simulink model "uavPackageDelivery_3UAV_photo3D_test"  (R2026a)
settings: Solver=VariableStepAuto  StopTime=20  FixedStep=.005  EnableMultiTasking=on
undefined symbols (not defined in the file or in its folder): baseMission, Newton, oaMission, Raphson, uavIC_latLon, UAVSampleTime
libraries: robotcorelib x3, uavalgslib x3, robotalgslib x3, simulink x2
(part 1 of 2)
settings Model: DataDictionary=uavPackageDeliveryDataDict.sldd  ModifiedByFormat=The MathWorks, Inc.  PauseTimes=77  Creator=The MathWorks, Inc.  LastModifiedBy=The MathWorks, Inc.
settings OptimizationCC: DefaultUnderspecifiedDataType=single  PassReuseOutputArgsThreshold=0.0
settings DebuggingCC: ParameterPrecisionLossMsg=none
settings HardwareCC: ProdHWDeviceType=Generic->Unspecified (assume 32-bit Generic)
settings RTWCC: GenerateReport=on  LaunchReport=on

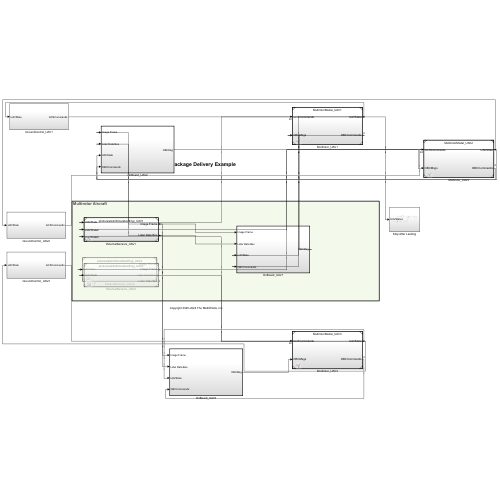
[thumbnail: Simulink's stored preview of the top-level diagram]
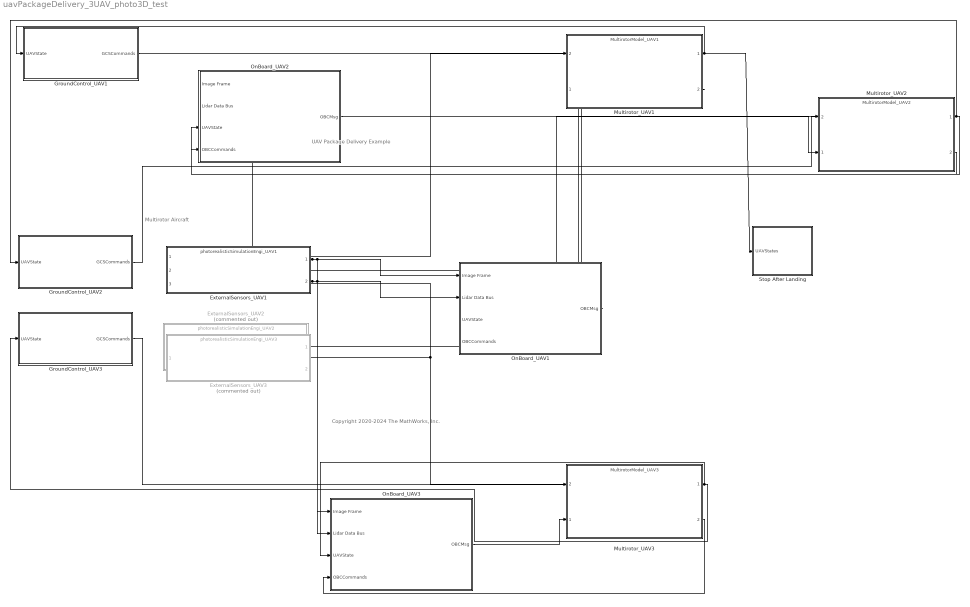
== system uavPackageDelivery_3UAV_photo3D_test ==
  note: Multirotor Aircraft
  note: UAV Package Delivery Example
  note: Copyright 2020-2024 The MathWorks, Inc.
  ExternalSensors_UAV1 : ModelReference  ModelNameDialog=photorealisticSimulationEngi_UAV1  SimulationMode=Normal  ModelReferenceVersion=12.27
  ExternalSensors_UAV2 : ModelReference  Commented=on  ModelNameDialog=photorealisticSimulationEngi_UAV2  SimulationMode=Normal  ModelReferenceVersion=12.1
  ExternalSensors_UAV3 : ModelReference  Commented=on  ModelNameDialog=photorealisticSimulationEngi_UAV3  SimulationMode=Normal  ModelReferenceVersion=12.1
  GroundControl_UAV1 : Subsystem
  GroundControl_UAV2 : Subsystem
  GroundControl_UAV3 : Subsystem
  Multirotor_UAV1 : ModelReference  ModelNameDialog=MultirotorModel_UAV1  SimulationMode=Normal  ModelReferenceVersion=13.15
      settings: PortSchema="{\"entries\":[{\"content\":{\"sides\":[{\"content\":{\"connectorIds\":[\"In2\",\"In1\"]},\"type\":\"ConnectorPlacement.EquallySpacedRectSide\",\"uuid\":\"abf53b88-b4c0-4cc3-bb4c-819ba68ade90\"},{\"content\":{\"connectorIds\":[\"Out1\",\"Out2\"],\"side\":\"RIGHT\"},\"type\":\"ConnectorPlacement.EquallySpacedRectSide\",\"uuid\":\"f1944fd3-3680-4558-bd6a-ffb0187ae725\"},{\"content\":{\"connectorIds\":[],\"side\":\"TOP\"},\"type\":\"ConnectorPlacement.EquallySpacedRectSide\",\"uuid\":\"7f686bac-a1b4-4e90-bc1f-e4dd6e8ae5c6\"}]},\"type\":\"ConnectorPlacement.EquallySpacedConnector\",\"uuid\":\"3f45c06a-90ee-44cf-add7-da13163a6845\"}],\"packageUris\":[\"http://schema.mathworks.com/mf0/Connector/19700101\"],\"version\":\"1.0\"}"
  Multirotor_UAV2 : ModelReference  ModelNameDialog=MultirotorModel_UAV2  SimulationMode=Normal  ModelReferenceVersion=13.16
      settings: PortSchema="{\"entries\":[{\"content\":{\"sides\":[{\"content\":{\"connectorIds\":[\"In2\",\"In1\"]},\"type\":\"ConnectorPlacement.EquallySpacedRectSide\",\"uuid\":\"abf53b88-b4c0-4cc3-bb4c-819ba68ade90\"},{\"content\":{\"connectorIds\":[\"Out1\",\"Out2\"],\"side\":\"RIGHT\"},\"type\":\"ConnectorPlacement.EquallySpacedRectSide\",\"uuid\":\"f1944fd3-3680-4558-bd6a-ffb0187ae725\"},{\"content\":{\"connectorIds\":[],\"side\":\"TOP\"},\"type\":\"ConnectorPlacement.EquallySpacedRectSide\",\"uuid\":\"7f686bac-a1b4-4e90-bc1f-e4dd6e8ae5c6\"}]},\"type\":\"ConnectorPlacement.EquallySpacedConnector\",\"uuid\":\"3f45c06a-90ee-44cf-add7-da13163a6845\"}],\"packageUris\":[\"http://schema.mathworks.com/mf0/Connector/19700101\"],\"version\":\"1.0\"}"
  Multirotor_UAV3 : ModelReference  ModelNameDialog=MultirotorModel_UAV3  SimulationMode=Normal  ModelReferenceVersion=13.16
      settings: PortSchema="{\"entries\":[{\"content\":{\"sides\":[{\"content\":{\"connectorIds\":[\"In2\",\"In1\"]},\"type\":\"ConnectorPlacement.EquallySpacedRectSide\",\"uuid\":\"abf53b88-b4c0-4cc3-bb4c-819ba68ade90\"},{\"content\":{\"connectorIds\":[\"Out1\",\"Out2\"],\"side\":\"RIGHT\"},\"type\":\"ConnectorPlacement.EquallySpacedRectSide\",\"uuid\":\"f1944fd3-3680-4558-bd6a-ffb0187ae725\"},{\"content\":{\"connectorIds\":[],\"side\":\"TOP\"},\"type\":\"ConnectorPlacement.EquallySpacedRectSide\",\"uuid\":\"7f686bac-a1b4-4e90-bc1f-e4dd6e8ae5c6\"}]},\"type\":\"ConnectorPlacement.EquallySpacedConnector\",\"uuid\":\"3f45c06a-90ee-44cf-add7-da13163a6845\"}],\"packageUris\":[\"http://schema.mathworks.com/mf0/Connector/19700101\"],\"version\":\"1.0\"}"
  OnBoard_UAV1 : Subsystem  TreatAsAtomicUnit=on
  OnBoard_UAV2 : Subsystem  TreatAsAtomicUnit=on
  OnBoard_UAV3 : Subsystem  TreatAsAtomicUnit=on
  Stop After Landing : Subsystem
  wires:
  GroundControl_UAV1/1(GCSCommands) -> Multirotor_UAV1/2
  Multirotor_UAV1/1 -> OnBoard_UAV1/3(UAVState), ExternalSensors_UAV1/1, GroundControl_UAV1/1(UAVState), Stop After Landing/1(UAVStates)
  Multirotor_UAV1/2 -> OnBoard_UAV1/4(OBCCommands)
  OnBoard_UAV1/1(OBCMsg) -> Multirotor_UAV1/1
  GroundControl_UAV2/1(GCSCommands) -> Multirotor_UAV2/2
  Multirotor_UAV2/1 -> ExternalSensors_UAV2/1, ExternalSensors_UAV1/2, GroundControl_UAV2/1(UAVState), OnBoard_UAV2/3(UAVState)
  Multirotor_UAV2/2 -> OnBoard_UAV2/4(OBCCommands)
  OnBoard_UAV2/1(OBCMsg) -> Multirotor_UAV2/1
  GroundControl_UAV3/1(GCSCommands) -> Multirotor_UAV3/2
  Multirotor_UAV3/1 -> ExternalSensors_UAV3/1, ExternalSensors_UAV1/3, GroundControl_UAV3/1(UAVState), OnBoard_UAV3/3(UAVState)
  Multirotor_UAV3/2 -> OnBoard_UAV3/4(OBCCommands)
  OnBoard_UAV3/1(OBCMsg) -> Multirotor_UAV3/1
  ExternalSensors_UAV1/1 -> OnBoard_UAV1/1(Image Frame), OnBoard_UAV3/1(Image Frame), OnBoard_UAV2/1(Image Frame)
  ExternalSensors_UAV1/2 -> OnBoard_UAV1/2("Lidar Data Bus "), OnBoard_UAV3/2("Lidar Data Bus "), OnBoard_UAV2/2("Lidar Data Bus ")

== system uavPackageDelivery_3UAV_photo3D_test/GroundControl_UAV1 ==
  UAVState : Inport  OutDataTypeStr=Bus: uavStateBus
  Get Flight Mission : Subsystem  Variant=on
  Rate Transition : RateTransition  OutPortSampleTime=UAVSampleTime*4
  GCSCommands : Outport
  wires:
  UAVState/1 -> Rate Transition/1
  Get Flight Mission/1("Mission ") -> GCSCommands/1
  Rate Transition/1 -> Get Flight Mission/1(UAVState)

== system uavPackageDelivery_3UAV_photo3D_test/GroundControl_UAV2 ==
  UAVState : Inport  OutDataTypeStr=Bus: uavStateBus
  Get Flight Mission : Subsystem  Variant=on
  Rate Transition : RateTransition  OutPortSampleTime=UAVSampleTime*4
  GCSCommands : Outport
  wires:
  UAVState/1 -> Rate Transition/1
  Get Flight Mission/1("Mission ") -> GCSCommands/1
  Rate Transition/1 -> Get Flight Mission/1(UAVState)

== system uavPackageDelivery_3UAV_photo3D_test/GroundControl_UAV3 ==
  UAVState : Inport  OutDataTypeStr=Bus: uavStateBus
  Get Flight Mission : Subsystem  Variant=on
  Rate Transition : RateTransition  OutPortSampleTime=UAVSampleTime*4
  GCSCommands : Outport
  wires:
  UAVState/1 -> Rate Transition/1
  Get Flight Mission/1("Mission ") -> GCSCommands/1
  Rate Transition/1 -> Get Flight Mission/1(UAVState)

== system uavPackageDelivery_3UAV_photo3D_test/OnBoard_UAV1 ==
  Image Frame : Inport
  "Lidar Data Bus " : Inport  Port=2
  UAVState : Inport  Port=3  OutDataTypeStr=Bus: uavStateBus  SampleTime=UAVSampleTime  BusOutputAsStruct=on
  OBCCommands : Inport  Port=4
  DataProcessing : Subsystem  Variant=on  PropagateVariantConditions=on
  Rate Transition : RateTransition  OutPortSampleTime=UAVSampleTime*4
  OBCMsg : Outport  OutDataTypeStr=single
  wires:
  Image Frame/1 -> DataProcessing/1(Image Frame)
  "Lidar Data Bus "/1 -> DataProcessing/2("Lidar Data Bus ")
  UAVState/1 -> DataProcessing/3(UAVState)
  OBCCommands/1 -> DataProcessing/4(OBCCommands)
  DataProcessing/1(OBCMsg) -> Rate Transition/1
  Rate Transition/1 -> OBCMsg/1

== system uavPackageDelivery_3UAV_photo3D_test/OnBoard_UAV2 ==
  Image Frame : Inport
  "Lidar Data Bus " : Inport  Port=2
  UAVState : Inport  Port=3  OutDataTypeStr=Bus: uavStateBus  SampleTime=UAVSampleTime  BusOutputAsStruct=on
  OBCCommands : Inport  Port=4
  DataProcessing : Subsystem  Variant=on  PropagateVariantConditions=on
  Rate Transition : RateTransition  OutPortSampleTime=UAVSampleTime*4
  OBCMsg : Outport  OutDataTypeStr=single
  wires:
  Image Frame/1 -> DataProcessing/1(Image Frame)
  "Lidar Data Bus "/1 -> DataProcessing/2("Lidar Data Bus ")
  UAVState/1 -> DataProcessing/3(UAVState)
  OBCCommands/1 -> DataProcessing/4(OBCCommands)
  DataProcessing/1(OBCMsg) -> Rate Transition/1
  Rate Transition/1 -> OBCMsg/1

== system uavPackageDelivery_3UAV_photo3D_test/OnBoard_UAV3 ==
  Image Frame : Inport
  "Lidar Data Bus " : Inport  Port=2
  UAVState : Inport  Port=3  OutDataTypeStr=Bus: uavStateBus  SampleTime=UAVSampleTime  BusOutputAsStruct=on
  OBCCommands : Inport  Port=4
  DataProcessing : Subsystem  Variant=on  PropagateVariantConditions=on
  Rate Transition : RateTransition  OutPortSampleTime=UAVSampleTime*4
  OBCMsg : Outport  OutDataTypeStr=single
  wires:
  Image Frame/1 -> DataProcessing/1(Image Frame)
  "Lidar Data Bus "/1 -> DataProcessing/2("Lidar Data Bus ")
  UAVState/1 -> DataProcessing/3(UAVState)
  OBCCommands/1 -> DataProcessing/4(OBCCommands)
  DataProcessing/1(OBCMsg) -> Rate Transition/1
  Rate Transition/1 -> OBCMsg/1

== system uavPackageDelivery_3UAV_photo3D_test/Stop After Landing ==
  UAVStates : Inport
  AND : Logic  IconShape=distinctive  AllPortsSameDT=off  OutDataTypeStr=boolean
  Bus Selector : BusSelector  OutputSignals=pos_vel.z
  Clock : Clock
  Landing height : simulink/Logic and Bit Operations/Compare To Constant  relop=>=  const=-0.6  OutDataTypeStr=boolean
  Minimum Simulation Time : simulink/Logic and Bit Operations/Compare To Constant  relop=>=  const=10  OutDataTypeStr=boolean
  Stop Simulation : Stop
  wires:
  UAVStates/1 -> Bus Selector/1
  Bus Selector/1 -> Landing height/1  "<z>"
  Clock/1 -> Minimum Simulation Time/1
  Minimum Simulation Time/1 -> AND/1
  Landing height/1 -> AND/2
  AND/1 -> Stop Simulation/1

== system uavPackageDelivery_3UAV_photo3D_test/GroundControl_UAV1/Get Flight Mission ==
  UAVState : Inport
  QGC : Subsystem  TreatAsAtomicUnit=on  SystemSampleTime=UAVSampleTime*4  VariantControl=useQGC==1
  noQGC : Subsystem  TreatAsAtomicUnit=on  SystemSampleTime=UAVSampleTime*4  VariantControl=useQGC==0
  "Mission " : Outport

== system uavPackageDelivery_3UAV_photo3D_test/GroundControl_UAV2/Get Flight Mission ==
  UAVState : Inport
  QGC : Subsystem  TreatAsAtomicUnit=on  SystemSampleTime=UAVSampleTime*4  VariantControl=useQGC==1
  noQGC : Subsystem  TreatAsAtomicUnit=on  SystemSampleTime=UAVSampleTime*4  VariantControl=useQGC==0
  "Mission " : Outport

== system uavPackageDelivery_3UAV_photo3D_test/GroundControl_UAV3/Get Flight Mission ==
  UAVState : Inport
  QGC : Subsystem  TreatAsAtomicUnit=on  SystemSampleTime=UAVSampleTime*4  VariantControl=useQGC==1
  noQGC : Subsystem  TreatAsAtomicUnit=on  SystemSampleTime=UAVSampleTime*4  VariantControl=useQGC==0
  "Mission " : Outport

== system uavPackageDelivery_3UAV_photo3D_test/OnBoard_UAV1/DataProcessing ==
  Image Frame : Inport
  "Lidar Data Bus " : Inport  Port=2
  UAVState : Inport  Port=3  OutDataTypeStr=Bus: uavStateBus  SampleTime=0.005  BusOutputAsStruct=on
  OBCCommands : Inport  Port=4
  NoSensorDataToProcess : Subsystem  VariantControl=isPhotoRealisticSim==0
  Process3DSensorData : Subsystem  VariantControl=(isPhotoRealisticSim ==1 || isPhotoRealisticSim ==2) && guidanceType == 3
  ProcessSensorData : Subsystem  VariantControl="(isPhotoRealisticSim ==1 || isPhotoRealisticSim ==2)  && guidanceType ~= 3"
  OBCMsg : Outport  OutDataTypeStr=single  SampleTime=0.005

== system uavPackageDelivery_3UAV_photo3D_test/OnBoard_UAV2/DataProcessing ==
  Image Frame : Inport
  "Lidar Data Bus " : Inport  Port=2
  UAVState : Inport  Port=3  OutDataTypeStr=Bus: uavStateBus  SampleTime=0.005  BusOutputAsStruct=on
  OBCCommands : Inport  Port=4
  NoSensorDataToProcess : Subsystem  VariantControl=isPhotoRealisticSim==0
  Process3DSensorData : Subsystem  VariantControl=(isPhotoRealisticSim ==1 || isPhotoRealisticSim ==2) && guidanceType == 3
  ProcessSensorData : Subsystem  VariantControl="(isPhotoRealisticSim ==1 || isPhotoRealisticSim ==2)  && guidanceType ~= 3"
  OBCMsg : Outport  OutDataTypeStr=single  SampleTime=0.005

== system uavPackageDelivery_3UAV_photo3D_test/OnBoard_UAV3/DataProcessing ==
  Image Frame : Inport
  "Lidar Data Bus " : Inport  Port=2
  UAVState : Inport  Port=3  OutDataTypeStr=Bus: uavStateBus  SampleTime=0.005  BusOutputAsStruct=on
  OBCCommands : Inport  Port=4
  NoSensorDataToProcess : Subsystem  VariantControl=isPhotoRealisticSim==0
  Process3DSensorData : Subsystem  VariantControl=(isPhotoRealisticSim ==1 || isPhotoRealisticSim ==2) && guidanceType == 3
  ProcessSensorData : Subsystem  VariantControl="(isPhotoRealisticSim ==1 || isPhotoRealisticSim ==2)  && guidanceType ~= 3"
  OBCMsg : Outport  OutDataTypeStr=single  SampleTime=0.005

== system uavPackageDelivery_3UAV_photo3D_test/GroundControl_UAV1/Get Flight Mission/QGC ==
  UAVState : Inport  OutDataTypeStr=Bus: uavStateBus
  Basline Mission : Constant  Value=baseMission  OutDataTypeStr=Bus: uavPathManagerBus  SampleTime=-1
  Create Mission for Path Manager : MATLAB Function  TreatAsAtomicUnit=on
  Delay : Delay  DelayLength=1
  MAVLink Interface : MATLABSystem  System=MAVLinkInterface  GCSPort=14550  MaxMissionLength=42  homeLatitude=uavIC_latLon(1)  homeLongitude=uavIC_latLon(2)
      mask Type: MAVLinkInterface
  Mission Items : Display
  Mission to Xe : Subsystem
  Mission : Outport  OutDataTypeStr=Bus: uavPathManagerBus
  wires:
  MAVLink Interface/3 -> Create Mission for Path Manager/2(isNew), Mission to Xe/Enable
  Basline Mission/1 -> Create Mission for Path Manager/1(baseMission)
  Mission to Xe/1(LTPMission) -> Create Mission for Path Manager/3(LTPMission)
  Create Mission for Path Manager/1(mission) -> Mission/1
  MAVLink Interface/1 -> Mission to Xe/1(QGCMission), Create Mission for Path Manager/4(qgcMission)
  Delay/1 -> MAVLink Interface/1
  UAVState/1 -> Delay/1
  MAVLink Interface/2 -> Mission Items/1

== system uavPackageDelivery_3UAV_photo3D_test/GroundControl_UAV1/Get Flight Mission/noQGC ==
  Variant Source : VariantSource  VariantControls={guidanceType==1, guidanceType==2 || guidanceType == 3}
  Waypoints : Constant  Value=baseMission  OutDataTypeStr=Bus: uavPathManagerBus  SampleTime=-1
  Waypoints1 : Constant  Value=oaMission  OutDataTypeStr=Bus: uavPathManagerBus  SampleTime=-1
  Mission : Outport
  wires:
  Waypoints/1 -> Variant Source/1
  Waypoints1/1 -> Variant Source/2
  Variant Source/1 -> Mission/1

== system uavPackageDelivery_3UAV_photo3D_test/GroundControl_UAV2/Get Flight Mission/QGC ==
  UAVState : Inport  OutDataTypeStr=Bus: uavStateBus
  Basline Mission : Constant  Value=baseMission  OutDataTypeStr=Bus: uavPathManagerBus  SampleTime=-1
  Create Mission for Path Manager : MATLAB Function  TreatAsAtomicUnit=on
  Delay : Delay  DelayLength=1
  MAVLink Interface : MATLABSystem  System=MAVLinkInterface  GCSPort=14550  MaxMissionLength=42  homeLatitude=uavIC_latLon(1)  homeLongitude=uavIC_latLon(2)
      mask Type: MAVLinkInterface
  Mission Items : Display
  Mission to Xe : Subsystem
  Mission : Outport  OutDataTypeStr=Bus: uavPathManagerBus
  wires:
  MAVLink Interface/3 -> Create Mission for Path Manager/2(isNew), Mission to Xe/Enable
  Basline Mission/1 -> Create Mission for Path Manager/1(baseMission)
  Mission to Xe/1(LTPMission) -> Create Mission for Path Manager/3(LTPMission)
  Create Mission for Path Manager/1(mission) -> Mission/1
  MAVLink Interface/1 -> Mission to Xe/1(QGCMission), Create Mission for Path Manager/4(qgcMission)
  Delay/1 -> MAVLink Interface/1
  UAVState/1 -> Delay/1
  MAVLink Interface/2 -> Mission Items/1

== system uavPackageDelivery_3UAV_photo3D_test/GroundControl_UAV2/Get Flight Mission/noQGC ==
  Variant Source : VariantSource  VariantControls={guidanceType==1, guidanceType==2 || guidanceType == 3}
  Waypoints : Constant  Value=baseMission  OutDataTypeStr=Bus: uavPathManagerBus  SampleTime=-1
  Waypoints1 : Constant  Value=oaMission  OutDataTypeStr=Bus: uavPathManagerBus  SampleTime=-1
  Mission : Outport
  wires:
  Waypoints/1 -> Variant Source/1
  Waypoints1/1 -> Variant Source/2
  Variant Source/1 -> Mission/1

== system uavPackageDelivery_3UAV_photo3D_test/GroundControl_UAV3/Get Flight Mission/QGC ==
  UAVState : Inport  OutDataTypeStr=Bus: uavStateBus
  Basline Mission : Constant  Value=baseMission  OutDataTypeStr=Bus: uavPathManagerBus  SampleTime=-1
  Create Mission for Path Manager : MATLAB Function  TreatAsAtomicUnit=on
  Delay : Delay  DelayLength=1
  MAVLink Interface : MATLABSystem  System=MAVLinkInterface  GCSPort=14550  MaxMissionLength=42  homeLatitude=uavIC_latLon(1)  homeLongitude=uavIC_latLon(2)
      mask Type: MAVLinkInterface
  Mission Items : Display
  Mission to Xe : Subsystem
  Mission : Outport  OutDataTypeStr=Bus: uavPathManagerBus
  wires:
  MAVLink Interface/3 -> Create Mission for Path Manager/2(isNew), Mission to Xe/Enable
  Basline Mission/1 -> Create Mission for Path Manager/1(baseMission)
  Mission to Xe/1(LTPMission) -> Create Mission for Path Manager/3(LTPMission)
  Create Mission for Path Manager/1(mission) -> Mission/1
  MAVLink Interface/1 -> Mission to Xe/1(QGCMission), Create Mission for Path Manager/4(qgcMission)
  Delay/1 -> MAVLink Interface/1
  UAVState/1 -> Delay/1
  MAVLink Interface/2 -> Mission Items/1

== system uavPackageDelivery_3UAV_photo3D_test/GroundControl_UAV3/Get Flight Mission/noQGC ==
  Variant Source : VariantSource  VariantControls={guidanceType==1, guidanceType==2 || guidanceType == 3}
  Waypoints : Constant  Value=baseMission  OutDataTypeStr=Bus: uavPathManagerBus  SampleTime=-1
  Waypoints1 : Constant  Value=oaMission  OutDataTypeStr=Bus: uavPathManagerBus  SampleTime=-1
  Mission : Outport
  wires:
  Waypoints/1 -> Variant Source/1
  Waypoints1/1 -> Variant Source/2
  Variant Source/1 -> Mission/1

== system uavPackageDelivery_3UAV_photo3D_test/OnBoard_UAV1/DataProcessing/NoSensorDataToProcess ==
  Image Frame : Inport
  "Lidar Data Bus " : Inport  Port=2
  UAVState : Inport  Port=3  OutDataTypeStr=Bus: uavStateBus  SampleTime=UAVSampleTime  BusOutputAsStruct=on
  OBCCommands : Inport  Port=4
  Ground : Ground
  Terminator{,1..3} (4 alike) : Terminator
  OBCMsg : Outport  OutDataTypeStr=single  SampleTime=UAVSampleTime
  wires:
  Ground/1 -> OBCMsg/1
  Image Frame/1 -> Terminator/1
  "Lidar Data Bus "/1 -> Terminator1/1
  UAVState/1 -> Terminator2/1
  OBCCommands/1 -> Terminator3/1

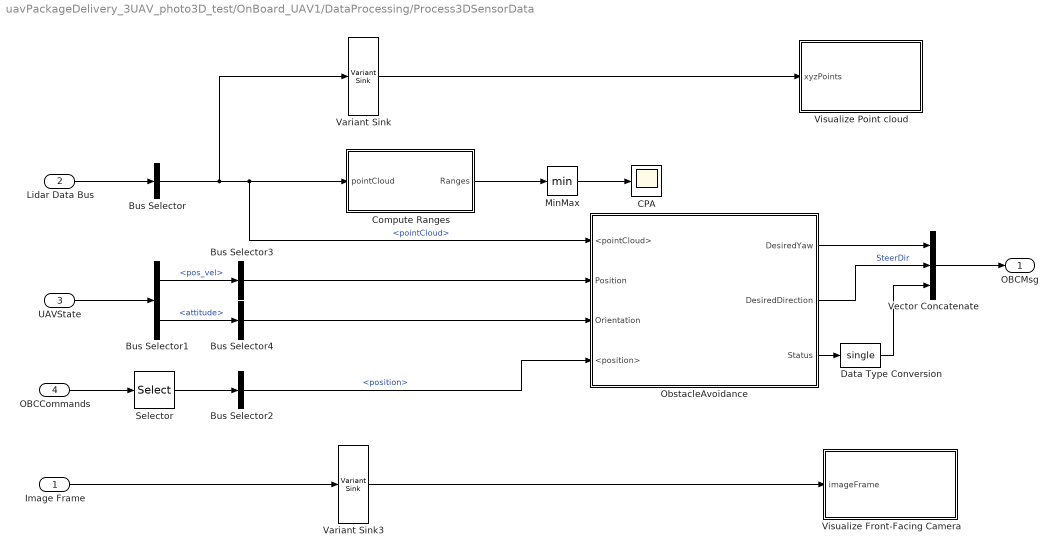
== system uavPackageDelivery_3UAV_photo3D_test/OnBoard_UAV1/DataProcessing/Process3DSensorData ==
  Image Frame : Inport
  "Lidar Data Bus " : Inport  Port=2  SampleTime=0.5
  UAVState : Inport  Port=3  OutDataTypeStr=Bus: uavStateBus  SampleTime=0.5  BusOutputAsStruct=on
  OBCCommands : Inport  Port=4  SampleTime=0.5
  Bus Selector : BusSelector  OutputSignals=pointCloud
  Bus Selector1 : BusSelector  OutputSignals=pos_vel,attitude
  Bus Selector2 : BusSelector  OutputSignals=position
  Bus Selector3 : BusSelector  OutputSignals=x,y,z  OutputAsBus=on
  Bus Selector4 : BusSelector  OutputSignals=yaw,pitch,roll  OutputAsBus=on
  CPA : Scope
      settings: TimeSpan=200  ActiveDisplayYMinimum=-1.62863  ActiveDisplayYMaximum=22.80719
  Compute Ranges : Subsystem
  Data Type Conversion : DataTypeConversion  OutDataTypeStr=single  SaturateOnIntegerOverflow=off  RndMeth=Floor
  MinMax : MinMax
  ObstacleAvoidance : Subsystem
  Selector : Selector  InputPortWidth=2  IndexOptions=Index vector (dialog)  Indices=[2]  OutputSizes=1
  Variant Sink : VariantSink  VariantControls={showLidarPointCloud ==1}
      settings: AllowZeroVariantControls=on
  Variant Sink3 : VariantSink  VariantControls={showVideoViewer == 1}
      settings: AllowZeroVariantControls=on
  Vector Concatenate : Concatenate  NumInputs=3
  Visualize Front-Facing Camera : MATLAB Function  TreatAsAtomicUnit=on
  Visualize Point cloud : MATLAB Function  StopFcn=|  TreatAsAtomicUnit=on
      | playerFigure = findall(groot,'type','figure','name','Point Cloud Player');
      | 
      | if ~isempty(playerFigure)
      |     playerFigure = playerFigure(end);
      |     if isvalid(playerFigure)
      |         close(playerFigure);
      |     end
      | end
  OBCMsg : Outport  OutDataTypeStr=single  SampleTime=0.005
  wires:
  Bus Selector/1 -> ObstacleAvoidance/1(<pointCloud>), Compute Ranges/1(pointCloud), Variant Sink/1  "<pointCloud>"
  Bus Selector1/2 -> Bus Selector4/1  "<attitude>"
  Variant Sink/1 -> Visualize Point cloud/1(xyzPoints)
  Selector/1 -> Bus Selector2/1
  MinMax/1 -> CPA/1
  Image Frame/1 -> Variant Sink3/1
  Bus Selector1/1 -> Bus Selector3/1  "<pos_vel>"
  UAVState/1 -> Bus Selector1/1
  "Lidar Data Bus "/1 -> Bus Selector/1
  Vector Concatenate/1 -> OBCMsg/1
  ObstacleAvoidance/1(DesiredYaw) -> Vector Concatenate/1
  Compute Ranges/1(Ranges) -> MinMax/1
  Bus Selector4/1 -> ObstacleAvoidance/3(Orientation)
  Bus Selector3/1 -> ObstacleAvoidance/2(Position)
  Bus Selector2/1 -> ObstacleAvoidance/4(<position>)  "<position>"
  ObstacleAvoidance/2(DesiredDirection) -> Vector Concatenate/2  "SteerDir"
  OBCCommands/1 -> Selector/1
  Variant Sink3/1 -> Visualize Front-Facing Camera/1(imageFrame)
  ObstacleAvoidance/3(Status) -> Data Type Conversion/1
  Data Type Conversion/1 -> Vector Concatenate/3

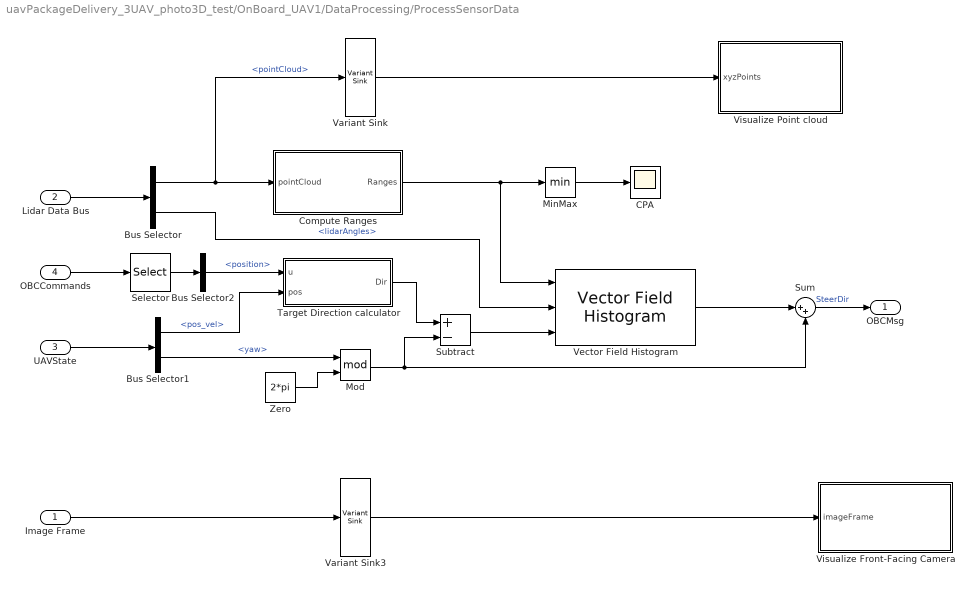
== system uavPackageDelivery_3UAV_photo3D_test/OnBoard_UAV1/DataProcessing/ProcessSensorData ==
  Image Frame : Inport
  "Lidar Data Bus " : Inport  Port=2  SampleTime=UAVSampleTime*10
  UAVState : Inport  Port=3  OutDataTypeStr=Bus: uavStateBus  SampleTime=UAVSampleTime*10  BusOutputAsStruct=on
  OBCCommands : Inport  Port=4  SampleTime=UAVSampleTime*10
  Bus Selector : BusSelector  OutputSignals=pointCloud,lidarAngles
  Bus Selector1 : BusSelector  OutputSignals=pos_vel,attitude.yaw
  Bus Selector2 : BusSelector  OutputSignals=position
  CPA : Scope
      settings: TimeSpan=200  ActiveDisplayYMinimum=3.83822  ActiveDisplayYMaximum=27.99117
  Compute Ranges : Subsystem
  MinMax : MinMax
  Mod : Math  Operator=mod
  Selector : Selector  InputPortWidth=2  IndexOptions=Index vector (dialog)  Indices=[2]  OutputSizes=1
  Subtract : Sum  Inputs=+-
  Sum : Sum  Inputs=|++  AccumDataTypeStr=single
  Target Direction calculator : MATLAB Function  TreatAsAtomicUnit=on
  Variant Sink : VariantSink  VariantControls={showLidarPointCloud ==1}
      settings: AllowZeroVariantControls=on
  Variant Sink3 : VariantSink  VariantControls={showVideoViewer == 1}
      settings: AllowZeroVariantControls=on
  Vector Field Histogram : robotalgslib/Vector Field Histogram  NumAngularSectors=360  DistanceLimits=[ 0 , 30 ]  HistogramThresholds=[ 5, 10 ]  RobotRadius=.5  SafetyDistance=0.65  MinTurningRadius=2  SimulateUsing=Code generation  TargetDirectionWeight=5  CurrentDirectionWeight=2  PreviousDirectionWeight=2
  Visualize Front-Facing Camera : MATLAB Function  TreatAsAtomicUnit=on
  Visualize Point cloud : MATLAB Function  StopFcn=|  TreatAsAtomicUnit=on
      | playerFigure = findall(groot,'type','figure','name','Point Cloud Player');
      | 
      | if ~isempty(playerFigure)
      |     playerFigure = playerFigure(end);
      |     if isvalid(playerFigure)
      |         close(playerFigure);
      |     end
      | end
  Zero : Constant  Value=2*pi  OutDataTypeStr=Inherit: Inherit via back propagation
  OBCMsg : Outport  OutDataTypeStr=single  SampleTime=0.005
  wires:
  UAVState/1 -> Bus Selector1/1
  Subtract/1 -> Vector Field Histogram/3
  Target Direction calculator/1(Dir) -> Subtract/1
  Bus Selector1/2 -> Mod/1  "<yaw>"
  Bus Selector2/1 -> Target Direction calculator/1(u)  "<position>"
  Bus Selector/2 -> Vector Field Histogram/2  "<lidarAngles>"
  "Lidar Data Bus "/1 -> Bus Selector/1
  Image Frame/1 -> Variant Sink3/1
  Zero/1 -> Mod/2
  Selector/1 -> Bus Selector2/1
  Compute Ranges/1(Ranges) -> MinMax/1, Vector Field Histogram/1
  Bus Selector/1 -> Compute Ranges/1(pointCloud), Variant Sink/1  "<pointCloud>"
  OBCCommands/1 -> Selector/1
  MinMax/1 -> CPA/1
  Variant Sink3/1 -> Visualize Front-Facing Camera/1(imageFrame)
  Sum/1 -> OBCMsg/1  "SteerDir"
  Bus Selector1/1 -> Target Direction calculator/2(pos)  "<pos_vel>"
  Variant Sink/1 -> Visualize Point cloud/1(xyzPoints)
  Mod/1 -> Sum/2, Subtract/2
  Vector Field Histogram/1 -> Sum/1

== system uavPackageDelivery_3UAV_photo3D_test/OnBoard_UAV2/DataProcessing/NoSensorDataToProcess ==
  Image Frame : Inport
  "Lidar Data Bus " : Inport  Port=2
  UAVState : Inport  Port=3  OutDataTypeStr=Bus: uavStateBus  SampleTime=UAVSampleTime  BusOutputAsStruct=on
  OBCCommands : Inport  Port=4
  Ground : Ground
  Terminator{,1..3} (4 alike) : Terminator
  OBCMsg : Outport  OutDataTypeStr=single  SampleTime=UAVSampleTime
  wires:
  Ground/1 -> OBCMsg/1
  Image Frame/1 -> Terminator/1
  "Lidar Data Bus "/1 -> Terminator1/1
  UAVState/1 -> Terminator2/1
  OBCCommands/1 -> Terminator3/1

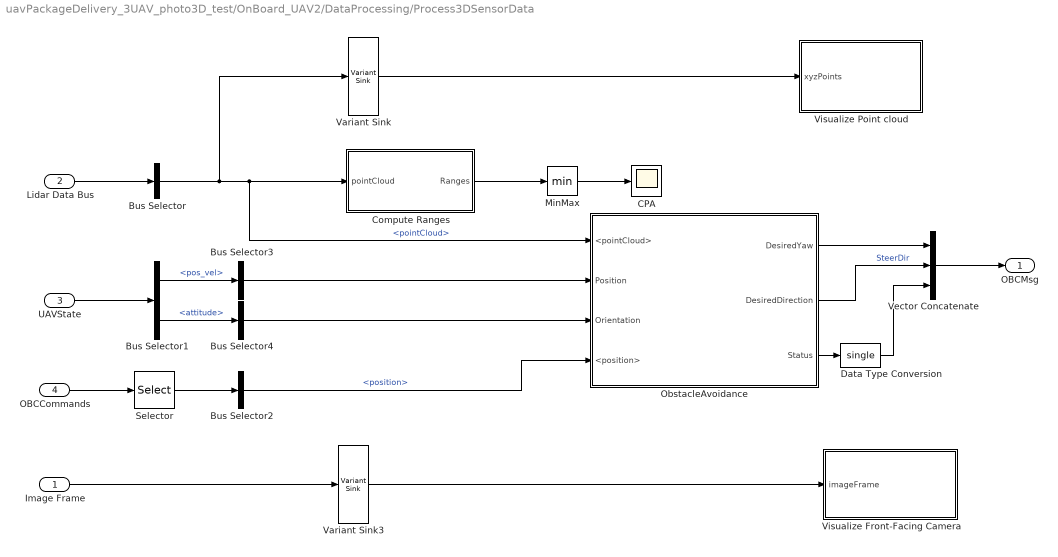
== system uavPackageDelivery_3UAV_photo3D_test/OnBoard_UAV2/DataProcessing/Process3DSensorData ==
  Image Frame : Inport
  "Lidar Data Bus " : Inport  Port=2  SampleTime=0.5
  UAVState : Inport  Port=3  OutDataTypeStr=Bus: uavStateBus  SampleTime=0.5  BusOutputAsStruct=on
  OBCCommands : Inport  Port=4  SampleTime=0.5
  Bus Selector : BusSelector  OutputSignals=pointCloud
  Bus Selector1 : BusSelector  OutputSignals=pos_vel,attitude
  Bus Selector2 : BusSelector  OutputSignals=position
  Bus Selector3 : BusSelector  OutputSignals=x,y,z  OutputAsBus=on
  Bus Selector4 : BusSelector  OutputSignals=yaw,pitch,roll  OutputAsBus=on
  CPA : Scope
      settings: TimeSpan=200  ActiveDisplayYMinimum=-1.62863  ActiveDisplayYMaximum=22.80719
  Compute Ranges : Subsystem
  Data Type Conversion : DataTypeConversion  OutDataTypeStr=single  SaturateOnIntegerOverflow=off  RndMeth=Floor
  MinMax : MinMax
  ObstacleAvoidance : Subsystem
  Selector : Selector  InputPortWidth=2  IndexOptions=Index vector (dialog)  Indices=[2]  OutputSizes=1
  Variant Sink : VariantSink  VariantControls={showLidarPointCloud ==1}
      settings: AllowZeroVariantControls=on
  Variant Sink3 : VariantSink  VariantControls={showVideoViewer == 1}
      settings: AllowZeroVariantControls=on
  Vector Concatenate : Concatenate  NumInputs=3
  Visualize Front-Facing Camera : MATLAB Function  TreatAsAtomicUnit=on
  Visualize Point cloud : MATLAB Function  StopFcn=|  TreatAsAtomicUnit=on
      | playerFigure = findall(groot,'type','figure','name','Point Cloud Player');
      | 
      | if ~isempty(playerFigure)
      |     playerFigure = playerFigure(end);
      |     if isvalid(playerFigure)
      |         close(playerFigure);
      |     end
      | end
  OBCMsg : Outport  OutDataTypeStr=single  SampleTime=0.005
  wires:
  Bus Selector/1 -> ObstacleAvoidance/1(<pointCloud>), Compute Ranges/1(pointCloud), Variant Sink/1  "<pointCloud>"
  Bus Selector1/2 -> Bus Selector4/1  "<attitude>"
  Variant Sink/1 -> Visualize Point cloud/1(xyzPoints)
  Selector/1 -> Bus Selector2/1
  MinMax/1 -> CPA/1
  Image Frame/1 -> Variant Sink3/1
  Bus Selector1/1 -> Bus Selector3/1  "<pos_vel>"
  UAVState/1 -> Bus Selector1/1
  "Lidar Data Bus "/1 -> Bus Selector/1
  Vector Concatenate/1 -> OBCMsg/1
  ObstacleAvoidance/1(DesiredYaw) -> Vector Concatenate/1
  Compute Ranges/1(Ranges) -> MinMax/1
  Bus Selector4/1 -> ObstacleAvoidance/3(Orientation)
  Bus Selector3/1 -> ObstacleAvoidance/2(Position)
  Bus Selector2/1 -> ObstacleAvoidance/4(<position>)  "<position>"
  ObstacleAvoidance/2(DesiredDirection) -> Vector Concatenate/2  "SteerDir"
  OBCCommands/1 -> Selector/1
  Variant Sink3/1 -> Visualize Front-Facing Camera/1(imageFrame)
  ObstacleAvoidance/3(Status) -> Data Type Conversion/1
  Data Type Conversion/1 -> Vector Concatenate/3

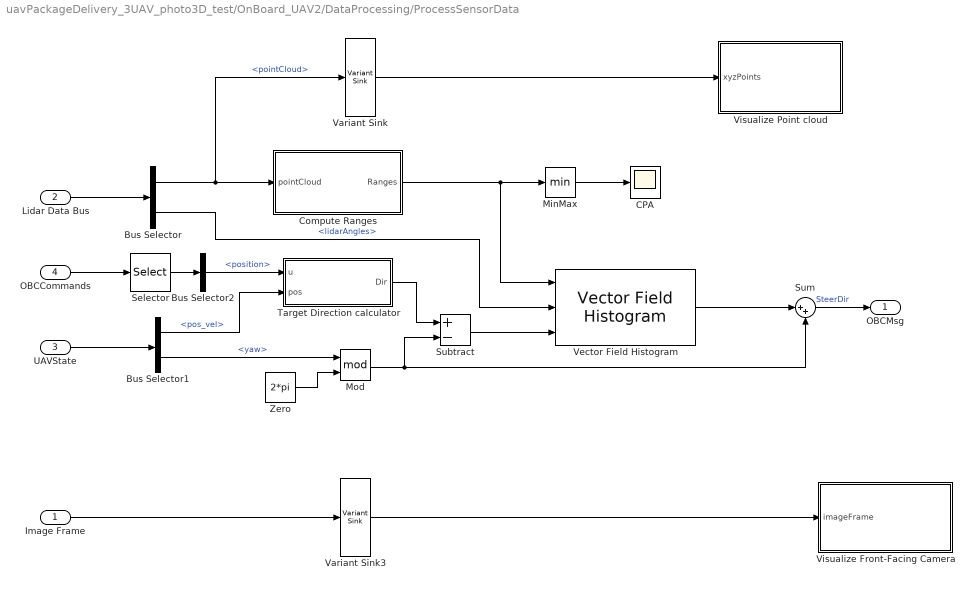
== system uavPackageDelivery_3UAV_photo3D_test/OnBoard_UAV2/DataProcessing/ProcessSensorData ==
  Image Frame : Inport
  "Lidar Data Bus " : Inport  Port=2  SampleTime=UAVSampleTime*10
  UAVState : Inport  Port=3  OutDataTypeStr=Bus: uavStateBus  SampleTime=UAVSampleTime*10  BusOutputAsStruct=on
  OBCCommands : Inport  Port=4  SampleTime=UAVSampleTime*10
  Bus Selector : BusSelector  OutputSignals=pointCloud,lidarAngles
  Bus Selector1 : BusSelector  OutputSignals=pos_vel,attitude.yaw
  Bus Selector2 : BusSelector  OutputSignals=position
  CPA : Scope
      settings: TimeSpan=200  ActiveDisplayYMinimum=3.83822  ActiveDisplayYMaximum=27.99117
  Compute Ranges : Subsystem
  MinMax : MinMax
  Mod : Math  Operator=mod
  Selector : Selector  InputPortWidth=2  IndexOptions=Index vector (dialog)  Indices=[2]  OutputSizes=1
  Subtract : Sum  Inputs=+-
  Sum : Sum  Inputs=|++  AccumDataTypeStr=single
  Target Direction calculator : MATLAB Function  TreatAsAtomicUnit=on
  Variant Sink : VariantSink  VariantControls={showLidarPointCloud ==1}
      settings: AllowZeroVariantControls=on
  Variant Sink3 : VariantSink  VariantControls={showVideoViewer == 1}
      settings: AllowZeroVariantControls=on
  Vector Field Histogram : robotalgslib/Vector Field Histogram  NumAngularSectors=360  DistanceLimits=[ 0 , 30 ]  HistogramThresholds=[ 5, 10 ]  RobotRadius=.5  SafetyDistance=0.65  MinTurningRadius=2  SimulateUsing=Code generation  TargetDirectionWeight=5  CurrentDirectionWeight=2  PreviousDirectionWeight=2
  Visualize Front-Facing Camera : MATLAB Function  TreatAsAtomicUnit=on
  Visualize Point cloud : MATLAB Function  StopFcn=|  TreatAsAtomicUnit=on
      | playerFigure = findall(groot,'type','figure','name','Point Cloud Player');
      | 
      | if ~isempty(playerFigure)
      |     playerFigure = playerFigure(end);
      |     if isvalid(playerFigure)
      |         close(playerFigure);
      |     end
      | end
  Zero : Constant  Value=2*pi  OutDataTypeStr=Inherit: Inherit via back propagation
  OBCMsg : Outport  OutDataTypeStr=single  SampleTime=0.005
  wires:
  UAVState/1 -> Bus Selector1/1
  Subtract/1 -> Vector Field Histogram/3
  Target Direction calculator/1(Dir) -> Subtract/1
  Bus Selector1/2 -> Mod/1  "<yaw>"
  Bus Selector2/1 -> Target Direction calculator/1(u)  "<position>"
  Bus Selector/2 -> Vector Field Histogram/2  "<lidarAngles>"
  "Lidar Data Bus "/1 -> Bus Selector/1
  Image Frame/1 -> Variant Sink3/1
  Zero/1 -> Mod/2
  Selector/1 -> Bus Selector2/1
  Compute Ranges/1(Ranges) -> MinMax/1, Vector Field Histogram/1
  Bus Selector/1 -> Compute Ranges/1(pointCloud), Variant Sink/1  "<pointCloud>"
  OBCCommands/1 -> Selector/1
  MinMax/1 -> CPA/1
  Variant Sink3/1 -> Visualize Front-Facing Camera/1(imageFrame)
  Sum/1 -> OBCMsg/1  "SteerDir"
  Bus Selector1/1 -> Target Direction calculator/2(pos)  "<pos_vel>"
  Variant Sink/1 -> Visualize Point cloud/1(xyzPoints)
  Mod/1 -> Sum/2, Subtract/2
  Vector Field Histogram/1 -> Sum/1

== system uavPackageDelivery_3UAV_photo3D_test/OnBoard_UAV3/DataProcessing/NoSensorDataToProcess ==
  Image Frame : Inport
  "Lidar Data Bus " : Inport  Port=2
  UAVState : Inport  Port=3  OutDataTypeStr=Bus: uavStateBus  SampleTime=UAVSampleTime  BusOutputAsStruct=on
  OBCCommands : Inport  Port=4
  Ground : Ground
  Terminator{,1..3} (4 alike) : Terminator
  OBCMsg : Outport  OutDataTypeStr=single  SampleTime=UAVSampleTime
  wires:
  Ground/1 -> OBCMsg/1
  Image Frame/1 -> Terminator/1
  "Lidar Data Bus "/1 -> Terminator1/1
  UAVState/1 -> Terminator2/1
  OBCCommands/1 -> Terminator3/1

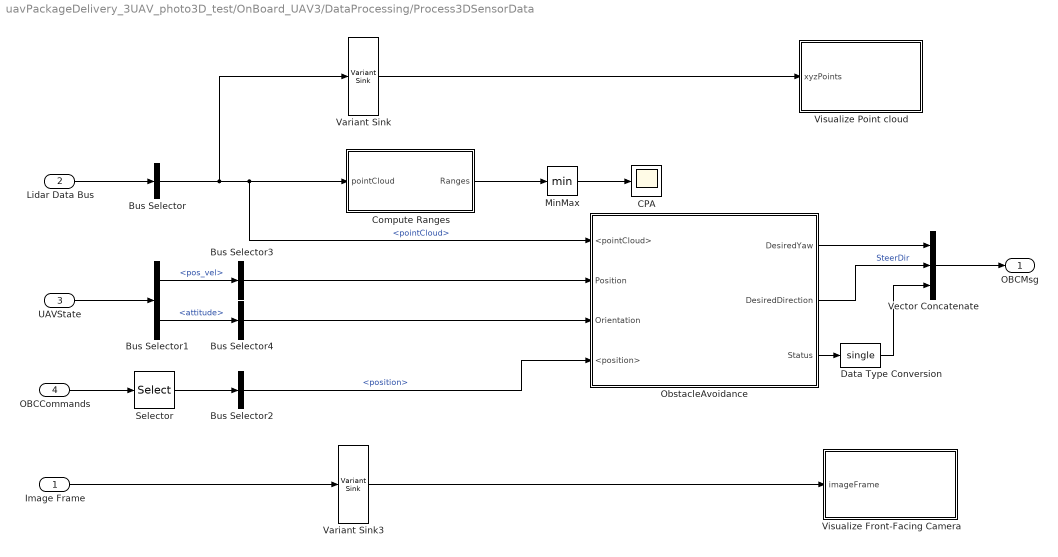
== system uavPackageDelivery_3UAV_photo3D_test/OnBoard_UAV3/DataProcessing/Process3DSensorData ==
  Image Frame : Inport
  "Lidar Data Bus " : Inport  Port=2  SampleTime=0.5
  UAVState : Inport  Port=3  OutDataTypeStr=Bus: uavStateBus  SampleTime=0.5  BusOutputAsStruct=on
  OBCCommands : Inport  Port=4  SampleTime=0.5
  Bus Selector : BusSelector  OutputSignals=pointCloud
  Bus Selector1 : BusSelector  OutputSignals=pos_vel,attitude
  Bus Selector2 : BusSelector  OutputSignals=position
  Bus Selector3 : BusSelector  OutputSignals=x,y,z  OutputAsBus=on
  Bus Selector4 : BusSelector  OutputSignals=yaw,pitch,roll  OutputAsBus=on
  CPA : Scope
      settings: TimeSpan=200  ActiveDisplayYMinimum=-1.62863  ActiveDisplayYMaximum=22.80719
  Compute Ranges : Subsystem
  Data Type Conversion : DataTypeConversion  OutDataTypeStr=single  SaturateOnIntegerOverflow=off  RndMeth=Floor
  MinMax : MinMax
  ObstacleAvoidance : Subsystem
  Selector : Selector  InputPortWidth=2  IndexOptions=Index vector (dialog)  Indices=[2]  OutputSizes=1
  Variant Sink : VariantSink  VariantControls={showLidarPointCloud ==1}
      settings: AllowZeroVariantControls=on
  Variant Sink3 : VariantSink  VariantControls={showVideoViewer == 1}
      settings: AllowZeroVariantControls=on
  Vector Concatenate : Concatenate  NumInputs=3
  Visualize Front-Facing Camera : MATLAB Function  TreatAsAtomicUnit=on
  Visualize Point cloud : MATLAB Function  StopFcn=|  TreatAsAtomicUnit=on
      | playerFigure = findall(groot,'type','figure','name','Point Cloud Player');
      | 
      | if ~isempty(playerFigure)
      |     playerFigure = playerFigure(end);
      |     if isvalid(playerFigure)
      |         close(playerFigure);
      |     end
      | end
  OBCMsg : Outport  OutDataTypeStr=single  SampleTime=0.005
  wires:
  Bus Selector/1 -> ObstacleAvoidance/1(<pointCloud>), Compute Ranges/1(pointCloud), Variant Sink/1  "<pointCloud>"
  Bus Selector1/2 -> Bus Selector4/1  "<attitude>"
  Variant Sink/1 -> Visualize Point cloud/1(xyzPoints)
  Selector/1 -> Bus Selector2/1
  MinMax/1 -> CPA/1
  Image Frame/1 -> Variant Sink3/1
  Bus Selector1/1 -> Bus Selector3/1  "<pos_vel>"
  UAVState/1 -> Bus Selector1/1
  "Lidar Data Bus "/1 -> Bus Selector/1
  Vector Concatenate/1 -> OBCMsg/1
  ObstacleAvoidance/1(DesiredYaw) -> Vector Concatenate/1
  Compute Ranges/1(Ranges) -> MinMax/1
  Bus Selector4/1 -> ObstacleAvoidance/3(Orientation)
  Bus Selector3/1 -> ObstacleAvoidance/2(Position)
  Bus Selector2/1 -> ObstacleAvoidance/4(<position>)  "<position>"
  ObstacleAvoidance/2(DesiredDirection) -> Vector Concatenate/2  "SteerDir"
  OBCCommands/1 -> Selector/1
  Variant Sink3/1 -> Visualize Front-Facing Camera/1(imageFrame)
  ObstacleAvoidance/3(Status) -> Data Type Conversion/1
  Data Type Conversion/1 -> Vector Concatenate/3

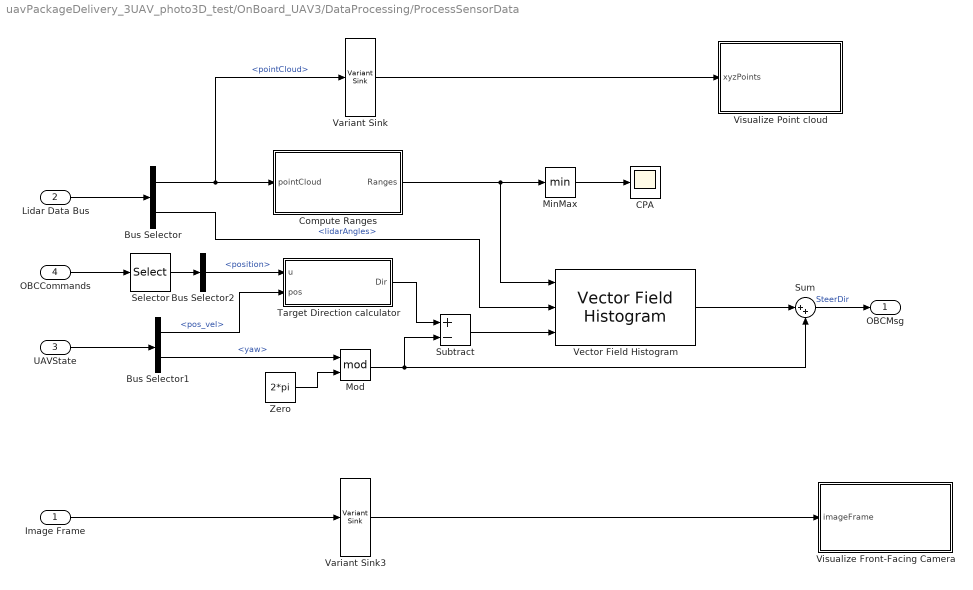
== system uavPackageDelivery_3UAV_photo3D_test/OnBoard_UAV3/DataProcessing/ProcessSensorData ==
  Image Frame : Inport
  "Lidar Data Bus " : Inport  Port=2  SampleTime=UAVSampleTime*10
  UAVState : Inport  Port=3  OutDataTypeStr=Bus: uavStateBus  SampleTime=UAVSampleTime*10  BusOutputAsStruct=on
  OBCCommands : Inport  Port=4  SampleTime=UAVSampleTime*10
  Bus Selector : BusSelector  OutputSignals=pointCloud,lidarAngles
  Bus Selector1 : BusSelector  OutputSignals=pos_vel,attitude.yaw
  Bus Selector2 : BusSelector  OutputSignals=position
  CPA : Scope
      settings: TimeSpan=200  ActiveDisplayYMinimum=3.83822  ActiveDisplayYMaximum=27.99117
  Compute Ranges : Subsystem
  MinMax : MinMax
  Mod : Math  Operator=mod
  Selector : Selector  InputPortWidth=2  IndexOptions=Index vector (dialog)  Indices=[2]  OutputSizes=1
  Subtract : Sum  Inputs=+-
  Sum : Sum  Inputs=|++  AccumDataTypeStr=single
  Target Direction calculator : MATLAB Function  TreatAsAtomicUnit=on
  Variant Sink : VariantSink  VariantControls={showLidarPointCloud ==1}
      settings: AllowZeroVariantControls=on
  Variant Sink3 : VariantSink  VariantControls={showVideoViewer == 1}
      settings: AllowZeroVariantControls=on
  Vector Field Histogram : robotalgslib/Vector Field Histogram  NumAngularSectors=360  DistanceLimits=[ 0 , 30 ]  HistogramThresholds=[ 5, 10 ]  RobotRadius=.5  SafetyDistance=0.65  MinTurningRadius=2  SimulateUsing=Code generation  TargetDirectionWeight=5  CurrentDirectionWeight=2  PreviousDirectionWeight=2
  Visualize Front-Facing Camera : MATLAB Function  TreatAsAtomicUnit=on
  Visualize Point cloud : MATLAB Function  StopFcn=|  TreatAsAtomicUnit=on
      | playerFigure = findall(groot,'type','figure','name','Point Cloud Player');
      | 
      | if ~isempty(playerFigure)
      |     playerFigure = playerFigure(end);
      |     if isvalid(playerFigure)
      |         close(playerFigure);
      |     end
      | end
  Zero : Constant  Value=2*pi  OutDataTypeStr=Inherit: Inherit via back propagation
  OBCMsg : Outport  OutDataTypeStr=single  SampleTime=0.005
  wires:
  UAVState/1 -> Bus Selector1/1
  Subtract/1 -> Vector Field Histogram/3
  Target Direction calculator/1(Dir) -> Subtract/1
  Bus Selector1/2 -> Mod/1  "<yaw>"
  Bus Selector2/1 -> Target Direction calculator/1(u)  "<position>"
  Bus Selector/2 -> Vector Field Histogram/2  "<lidarAngles>"
  "Lidar Data Bus "/1 -> Bus Selector/1
  Image Frame/1 -> Variant Sink3/1
  Zero/1 -> Mod/2
  Selector/1 -> Bus Selector2/1
  Compute Ranges/1(Ranges) -> MinMax/1, Vector Field Histogram/1
  Bus Selector/1 -> Compute Ranges/1(pointCloud), Variant Sink/1  "<pointCloud>"
  OBCCommands/1 -> Selector/1
  MinMax/1 -> CPA/1
  Variant Sink3/1 -> Visualize Front-Facing Camera/1(imageFrame)
  Sum/1 -> OBCMsg/1  "SteerDir"
  Bus Selector1/1 -> Target Direction calculator/2(pos)  "<pos_vel>"
  Variant Sink/1 -> Visualize Point cloud/1(xyzPoints)
  Mod/1 -> Sum/2, Subtract/2
  Vector Field Histogram/1 -> Sum/1

== system uavPackageDelivery_3UAV_photo3D_test/GroundControl_UAV1/Get Flight Mission/QGC/Mission to Xe ==
  QGCMission : Inport
  Enable : EnablePort
  For Each Subsystem : Subsystem  TreatAsAtomicUnit=on
  MATLAB Function : MATLAB Function  TreatAsAtomicUnit=on
  Transpose : Math  Operator=transpose
  LTPMission : Outport
  wires:
  For Each Subsystem/1(Xe) -> Transpose/1
  MATLAB Function/1(waypoints) -> For Each Subsystem/1(latLon)
  QGCMission/1 -> MATLAB Function/1(mission)
  Transpose/1 -> LTPMission/1

== system uavPackageDelivery_3UAV_photo3D_test/GroundControl_UAV2/Get Flight Mission/QGC/Mission to Xe ==
  QGCMission : Inport
  Enable : EnablePort
  For Each Subsystem : Subsystem  TreatAsAtomicUnit=on
  MATLAB Function : MATLAB Function  TreatAsAtomicUnit=on
  Transpose : Math  Operator=transpose
  LTPMission : Outport
  wires:
  For Each Subsystem/1(Xe) -> Transpose/1
  MATLAB Function/1(waypoints) -> For Each Subsystem/1(latLon)
  QGCMission/1 -> MATLAB Function/1(mission)
  Transpose/1 -> LTPMission/1

== system uavPackageDelivery_3UAV_photo3D_test/GroundControl_UAV3/Get Flight Mission/QGC/Mission to Xe ==
  QGCMission : Inport
  Enable : EnablePort
  For Each Subsystem : Subsystem  TreatAsAtomicUnit=on
  MATLAB Function : MATLAB Function  TreatAsAtomicUnit=on
  Transpose : Math  Operator=transpose
  LTPMission : Outport
  wires:
  For Each Subsystem/1(Xe) -> Transpose/1
  MATLAB Function/1(waypoints) -> For Each Subsystem/1(latLon)
  QGCMission/1 -> MATLAB Function/1(mission)
  Transpose/1 -> LTPMission/1

== system uavPackageDelivery_3UAV_photo3D_test/OnBoard_UAV1/DataProcessing/Process3DSensorData/Compute Ranges ==
  pointCloud : Inport
  For Each Subsystem1 : Subsystem  TreatAsAtomicUnit=on
  Reshape1 : Reshape  OutputDimensions=1083
  Ranges : Outport
  wires:
  For Each Subsystem1/1(Out1) -> Reshape1/1
  pointCloud/1 -> For Each Subsystem1/1(In1)
  Reshape1/1 -> Ranges/1

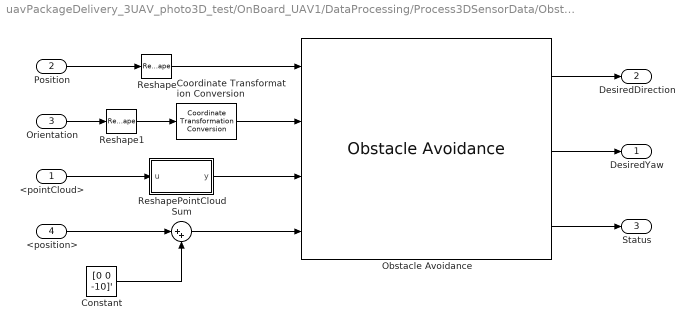
== system uavPackageDelivery_3UAV_photo3D_test/OnBoard_UAV1/DataProcessing/Process3DSensorData/ObstacleAvoidance ==
  <pointCloud> : Inport
  Position : Inport  Port=2
  Orientation : Inport  Port=3
  <position> : Inport  Port=4
  Constant : Constant  Value=[0 0 -10]'  VectorParams1D=off  OutDataTypeStr=single
  Coordinate Transformation Conversion : robotcorelib/Coordinate Transformation Conversion  InputRepresentation=Euler Angles  InputEulerSequence=ZYX  ShowTrVecInputPort=on  OutputRepresentation=Quaternion  OutputEulerSequence=ZYX  ShowTrVecOutputPort=on  SimulateUsing=Code generation
  Obstacle Avoidance : uavalgslib/Obstacle Avoidance  DistanceLimits=[ 0.2, 30 ]  HorizontalSensorFOV=[ -180, 180 ]  VerticalSensorFOV=[ -20, 20 ]  SensorLocation=[ 0, 0, -0.4 ]  SensorOrientation=[ 180, 0, 0 ]  VehicleRadius=0.5  SafetyDistance=0.75  SimulateUsing=Code generation  HistRes=5  WindowSize=1  HistogramThreshold=1  MaxAge=5  TargetDirectionWeight=3  CurrentDirectionWeight=1  PreviousDirectionWeight=2
  Reshape : Reshape  OutputDimensionality=Column vector (2-D)
  Reshape1 : Reshape  OutputDimensionality=Column vector (2-D)
  ReshapePointCloud : MATLAB Function  TreatAsAtomicUnit=on
  Sum : Sum  Inputs=|++
  DesiredYaw : Outport
  DesiredDirection : Outport  Port=2
  Status : Outport  Port=3
  wires:
  Obstacle Avoidance/1 -> DesiredDirection/1
  Obstacle Avoidance/3 -> Status/1
  <pointCloud>/1 -> ReshapePointCloud/1(u)
  Obstacle Avoidance/2 -> DesiredYaw/1
  Position/1 -> Reshape/1
  <position>/1 -> Sum/1
  Orientation/1 -> Reshape1/1
  Reshape/1 -> Obstacle Avoidance/1
  Reshape1/1 -> Coordinate Transformation Conversion/1
  ReshapePointCloud/1(y) -> Obstacle Avoidance/3
  Sum/1 -> Obstacle Avoidance/4
  Constant/1 -> Sum/2
  Coordinate Transformation Conversion/1 -> Obstacle Avoidance/2

== system uavPackageDelivery_3UAV_photo3D_test/OnBoard_UAV1/DataProcessing/ProcessSensorData/Compute Ranges ==
  pointCloud : Inport
  For Each Subsystem : Subsystem  TreatAsAtomicUnit=on
  Reshape : Reshape  OutputDimensionality=Customize  OutputDimensions=[1083 3]
  Reshape1 : Reshape  OutputDimensions=1083
  Selector1 : Selector  NumberOfDimensions=3  InputPortWidth=3  IndexOptions=Index vector (dialog),Select all,Select all  Indices=16,1,1  OutputSizes=1,1,1
  Ranges : Outport
  wires:
  For Each Subsystem/1(Out1) -> Reshape1/1
  Selector1/1 -> Reshape/1
  pointCloud/1 -> Selector1/1
  Reshape/1 -> For Each Subsystem/1(In1)
  Reshape1/1 -> Ranges/1

== system uavPackageDelivery_3UAV_photo3D_test/OnBoard_UAV2/DataProcessing/Process3DSensorData/Compute Ranges ==
  pointCloud : Inport
  For Each Subsystem1 : Subsystem  TreatAsAtomicUnit=on
  Reshape1 : Reshape  OutputDimensions=1083
  Ranges : Outport
  wires:
  For Each Subsystem1/1(Out1) -> Reshape1/1
  pointCloud/1 -> For Each Subsystem1/1(In1)
  Reshape1/1 -> Ranges/1

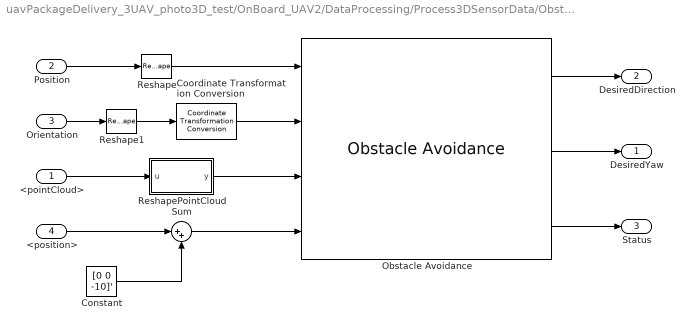
== system uavPackageDelivery_3UAV_photo3D_test/OnBoard_UAV2/DataProcessing/Process3DSensorData/ObstacleAvoidance ==
  <pointCloud> : Inport
  Position : Inport  Port=2
  Orientation : Inport  Port=3
  <position> : Inport  Port=4
  Constant : Constant  Value=[0 0 -10]'  VectorParams1D=off  OutDataTypeStr=single
  Coordinate Transformation Conversion : robotcorelib/Coordinate Transformation Conversion  InputRepresentation=Euler Angles  InputEulerSequence=ZYX  ShowTrVecInputPort=on  OutputRepresentation=Quaternion  OutputEulerSequence=ZYX  ShowTrVecOutputPort=on  SimulateUsing=Code generation
  Obstacle Avoidance : uavalgslib/Obstacle Avoidance  DistanceLimits=[ 0.2, 30 ]  HorizontalSensorFOV=[ -180, 180 ]  VerticalSensorFOV=[ -20, 20 ]  SensorLocation=[ 0, 0, -0.4 ]  SensorOrientation=[ 180, 0, 0 ]  VehicleRadius=0.5  SafetyDistance=0.75  SimulateUsing=Code generation  HistRes=5  WindowSize=1  HistogramThreshold=1  MaxAge=5  TargetDirectionWeight=3  CurrentDirectionWeight=1  PreviousDirectionWeight=2
  Reshape : Reshape  OutputDimensionality=Column vector (2-D)
  Reshape1 : Reshape  OutputDimensionality=Column vector (2-D)
  ReshapePointCloud : MATLAB Function  TreatAsAtomicUnit=on
  Sum : Sum  Inputs=|++
  DesiredYaw : Outport
  DesiredDirection : Outport  Port=2
  Status : Outport  Port=3
  wires:
  Obstacle Avoidance/1 -> DesiredDirection/1
  Obstacle Avoidance/3 -> Status/1
  <pointCloud>/1 -> ReshapePointCloud/1(u)
  Obstacle Avoidance/2 -> DesiredYaw/1
  Position/1 -> Reshape/1
  <position>/1 -> Sum/1
  Orientation/1 -> Reshape1/1
  Reshape/1 -> Obstacle Avoidance/1
  Reshape1/1 -> Coordinate Transformation Conversion/1
  ReshapePointCloud/1(y) -> Obstacle Avoidance/3
  Sum/1 -> Obstacle Avoidance/4
  Constant/1 -> Sum/2
  Coordinate Transformation Conversion/1 -> Obstacle Avoidance/2

== system uavPackageDelivery_3UAV_photo3D_test/OnBoard_UAV2/DataProcessing/ProcessSensorData/Compute Ranges ==
  pointCloud : Inport
  For Each Subsystem : Subsystem  TreatAsAtomicUnit=on
  Reshape : Reshape  OutputDimensionality=Customize  OutputDimensions=[1083 3]
  Reshape1 : Reshape  OutputDimensions=1083
  Selector1 : Selector  NumberOfDimensions=3  InputPortWidth=3  IndexOptions=Index vector (dialog),Select all,Select all  Indices=16,1,1  OutputSizes=1,1,1
  Ranges : Outport
  wires:
  For Each Subsystem/1(Out1) -> Reshape1/1
  Selector1/1 -> Reshape/1
  pointCloud/1 -> Selector1/1
  Reshape/1 -> For Each Subsystem/1(In1)
  Reshape1/1 -> Ranges/1

== system uavPackageDelivery_3UAV_photo3D_test/OnBoard_UAV3/DataProcessing/Process3DSensorData/Compute Ranges ==
  pointCloud : Inport
  For Each Subsystem1 : Subsystem  TreatAsAtomicUnit=on
  Reshape1 : Reshape  OutputDimensions=1083
  Ranges : Outport
  wires:
  For Each Subsystem1/1(Out1) -> Reshape1/1
  pointCloud/1 -> For Each Subsystem1/1(In1)
  Reshape1/1 -> Ranges/1

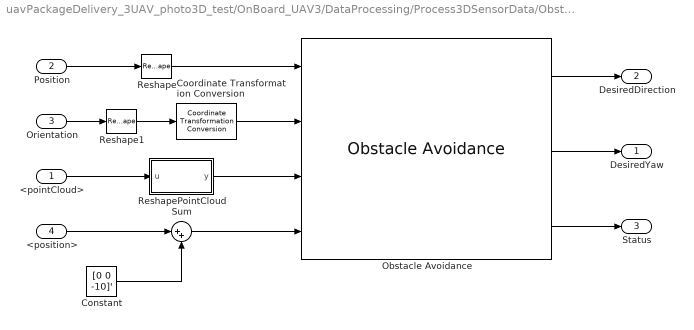
== system uavPackageDelivery_3UAV_photo3D_test/OnBoard_UAV3/DataProcessing/Process3DSensorData/ObstacleAvoidance ==
  <pointCloud> : Inport
  Position : Inport  Port=2
  Orientation : Inport  Port=3
  <position> : Inport  Port=4
  Constant : Constant  Value=[0 0 -10]'  VectorParams1D=off  OutDataTypeStr=single
  Coordinate Transformation Conversion : robotcorelib/Coordinate Transformation Conversion  InputRepresentation=Euler Angles  InputEulerSequence=ZYX  ShowTrVecInputPort=on  OutputRepresentation=Quaternion  OutputEulerSequence=ZYX  ShowTrVecOutputPort=on  SimulateUsing=Code generation
  Obstacle Avoidance : uavalgslib/Obstacle Avoidance  DistanceLimits=[ 0.2, 30 ]  HorizontalSensorFOV=[ -180, 180 ]  VerticalSensorFOV=[ -20, 20 ]  SensorLocation=[ 0, 0, -0.4 ]  SensorOrientation=[ 180, 0, 0 ]  VehicleRadius=0.5  SafetyDistance=0.75  SimulateUsing=Code generation  HistRes=5  WindowSize=1  HistogramThreshold=1  MaxAge=5  TargetDirectionWeight=3  CurrentDirectionWeight=1  PreviousDirectionWeight=2
  Reshape : Reshape  OutputDimensionality=Column vector (2-D)
  Reshape1 : Reshape  OutputDimensionality=Column vector (2-D)
  ReshapePointCloud : MATLAB Function  TreatAsAtomicUnit=on
  Sum : Sum  Inputs=|++
  DesiredYaw : Outport
  DesiredDirection : Outport  Port=2
  Status : Outport  Port=3
  wires:
  Obstacle Avoidance/1 -> DesiredDirection/1
  Obstacle Avoidance/3 -> Status/1
  <pointCloud>/1 -> ReshapePointCloud/1(u)
  Obstacle Avoidance/2 -> DesiredYaw/1
  Position/1 -> Reshape/1
  <position>/1 -> Sum/1
  Orientation/1 -> Reshape1/1
  Reshape/1 -> Obstacle Avoidance/1
  Reshape1/1 -> Coordinate Transformation Conversion/1
  ReshapePointCloud/1(y) -> Obstacle Avoidance/3
  Sum/1 -> Obstacle Avoidance/4
  Constant/1 -> Sum/2
  Coordinate Transformation Conversion/1 -> Obstacle Avoidance/2

== system uavPackageDelivery_3UAV_photo3D_test/OnBoard_UAV3/DataProcessing/ProcessSensorData/Compute Ranges ==
  pointCloud : Inport
  For Each Subsystem : Subsystem  TreatAsAtomicUnit=on
  Reshape : Reshape  OutputDimensionality=Customize  OutputDimensions=[1083 3]
  Reshape1 : Reshape  OutputDimensions=1083
  Selector1 : Selector  NumberOfDimensions=3  InputPortWidth=3  IndexOptions=Index vector (dialog),Select all,Select all  Indices=16,1,1  OutputSizes=1,1,1
  Ranges : Outport
  wires:
  For Each Subsystem/1(Out1) -> Reshape1/1
  Selector1/1 -> Reshape/1
  pointCloud/1 -> Selector1/1
  Reshape/1 -> For Each Subsystem/1(In1)
  Reshape1/1 -> Ranges/1

== system uavPackageDelivery_3UAV_photo3D_test/GroundControl_UAV1/Get Flight Mission/QGC/Mission to Xe/For Each Subsystem ==
  latLon : Inport  Partition=on  PartitionDimension=1  PartitionWidth=1  PartitionOffset=0
  Constant : Constant  Value=0  OutDataTypeStr=double
  Data Type Conversion : DataTypeConversion  OutDataTypeStr=single  SaturateOnIntegerOverflow=off  RndMeth=Floor
  Data Type Conversion1 : DataTypeConversion  OutDataTypeStr=double  SaturateOnIntegerOverflow=off  RndMeth=Floor
  Data Type Conversion2 : DataTypeConversion  OutDataTypeStr=double  SaturateOnIntegerOverflow=off  RndMeth=Floor
  Demux : Demux  Outputs=[2 1]
  For Each : ForEach  DisableCoverage=on
  LLA to Flat Earth : LLA2Flat  R=6378137  LL0=uavIC_latLon
  Xe : Outport  ConcatenationDimension=2
  wires:
  LLA to Flat Earth/1 -> Data Type Conversion/1
  Demux/2 -> Data Type Conversion2/1
  Demux/1 -> Data Type Conversion1/1
  latLon/1 -> Demux/1
  Constant/1 -> LLA to Flat Earth/3
  Data Type Conversion/1 -> Xe/1
  Data Type Conversion1/1 -> LLA to Flat Earth/1
  Data Type Conversion2/1 -> LLA to Flat Earth/2

== system uavPackageDelivery_3UAV_photo3D_test/GroundControl_UAV2/Get Flight Mission/QGC/Mission to Xe/For Each Subsystem ==
  latLon : Inport  Partition=on  PartitionDimension=1  PartitionWidth=1  PartitionOffset=0
  Constant : Constant  Value=0  OutDataTypeStr=double
  Data Type Conversion : DataTypeConversion  OutDataTypeStr=single  SaturateOnIntegerOverflow=off  RndMeth=Floor
  Data Type Conversion1 : DataTypeConversion  OutDataTypeStr=double  SaturateOnIntegerOverflow=off  RndMeth=Floor
  Data Type Conversion2 : DataTypeConversion  OutDataTypeStr=double  SaturateOnIntegerOverflow=off  RndMeth=Floor
  Demux : Demux  Outputs=[2 1]
  For Each : ForEach  DisableCoverage=on
  LLA to Flat Earth : LLA2Flat  R=6378137  LL0=uavIC_latLon
  Xe : Outport  ConcatenationDimension=2
  wires:
  LLA to Flat Earth/1 -> Data Type Conversion/1
  Demux/2 -> Data Type Conversion2/1
  Demux/1 -> Data Type Conversion1/1
  latLon/1 -> Demux/1
  Constant/1 -> LLA to Flat Earth/3
  Data Type Conversion/1 -> Xe/1
  Data Type Conversion1/1 -> LLA to Flat Earth/1
  Data Type Conversion2/1 -> LLA to Flat Earth/2

== system uavPackageDelivery_3UAV_photo3D_test/GroundControl_UAV3/Get Flight Mission/QGC/Mission to Xe/For Each Subsystem ==
  latLon : Inport  Partition=on  PartitionDimension=1  PartitionWidth=1  PartitionOffset=0
  Constant : Constant  Value=0  OutDataTypeStr=double
  Data Type Conversion : DataTypeConversion  OutDataTypeStr=single  SaturateOnIntegerOverflow=off  RndMeth=Floor
  Data Type Conversion1 : DataTypeConversion  OutDataTypeStr=double  SaturateOnIntegerOverflow=off  RndMeth=Floor
  Data Type Conversion2 : DataTypeConversion  OutDataTypeStr=double  SaturateOnIntegerOverflow=off  RndMeth=Floor
  Demux : Demux  Outputs=[2 1]
  For Each : ForEach  DisableCoverage=on
  LLA to Flat Earth : LLA2Flat  R=6378137  LL0=uavIC_latLon
  Xe : Outport  ConcatenationDimension=2
  wires:
  LLA to Flat Earth/1 -> Data Type Conversion/1
  Demux/2 -> Data Type Conversion2/1
  Demux/1 -> Data Type Conversion1/1
  latLon/1 -> Demux/1
  Constant/1 -> LLA to Flat Earth/3
  Data Type Conversion/1 -> Xe/1
  Data Type Conversion1/1 -> LLA to Flat Earth/1
  Data Type Conversion2/1 -> LLA to Flat Earth/2

== system uavPackageDelivery_3UAV_photo3D_test/OnBoard_UAV1/DataProcessing/Process3DSensorData/Compute Ranges/For Each Subsystem1 ==
  In1 : Inport  Partition=on  PartitionDimension=1  PartitionWidth=1  PartitionOffset=0
  For Each Horizontal Slice : ForEach  DisableCoverage=on
  Process each Horizontal Slice : Subsystem  TreatAsAtomicUnit=on
  Reshape : Reshape
  Out1 : Outport  ConcatenationDimension=1
  wires:
  In1/1 -> Process each Horizontal Slice/1(pointCloud)
  Process each Horizontal Slice/1(Out1) -> Reshape/1
  Reshape/1 -> Out1/1
